simulink model "helicopter"  (R2024b)
settings: Solver=VariableStepAuto  StartTime=0.0  StopTime=60  RelTol=1e-3
InitFcn:
  | % run(fullfile(".\C:\Users\omar_\OneDrive - Imperial College London\EIE Year 4\FYP\model\controllers\controller_top"));
  | % run(fullfile(".\C:\Users\omar_\OneDrive - Imperial College London\EIE Year 4\FYP\model\helicopter_functions\R"));
  | % run(fullfile(".\C:\Users\omar_\OneDrive - Imperial College London\EIE Year 4\FYP\model\helicopter_functions\R_inv"));
  | % run(fullfile(".\C:\Users\omar_\OneDrive - Imperial College London\EIE Year 4\FYP\model\helicopter_functions\axial_thrust"));
  | % run(fullfile(".\C:\Users\omar_\OneDrive - Imperial College London\EIE Year 4\FYP\model\helicopter_functions\axial_thrust_bot"));
  | % run(fullfile(".\C:\Users\omar_\OneDrive - Imperial College London\EIE Year 4\FYP\model\helicopter_functions\axial_thrust_top"));
  | % run(fullfile(".\C:\Users\omar_\OneDrive - Imperial College London\EIE Year 4\FYP\model\helicopter_functions\body_update"));
  | % run(fullfile(".\C:\Users\omar_\OneDrive - Imperial College London\EIE Year 4\FYP\model\helicopter_functions\controller_top"));
  | % run(fullfile(".\C:\Users\omar_\OneDrive - Imperial College London\EIE Year 4\FYP\model\helicopter_functions\earth_update"));
  | % run(fullfile(".\C:\Users\omar_\OneDrive - Imperial College London\EIE Year 4\FYP\model\helicopter_functions\load_variables"));
  | % run(fullfile(".\C:\Users\omar_\OneDrive - Imperial College London\EIE Year 4\FYP\model\helicopter_functions\thrust_moments"));
  | % run(fullfile(".\C:\Users\omar_\OneDrive - Imperial College London\EIE Year 4\FYP\model\swash_plate\swash"));
  | % run(fullfile(".\C:\Users\omar_\OneDrive - Imperial College London\EIE Year 4\FYP\model\swash_plate\swash_height"));
  | rpm_top=300;
  | rpm_bot=300;
settings Model: Creator=omar_  LastModifiedBy=omar_
settings DataIOCC: ExternalInput=ext_sigs  LoadExternalInput=on

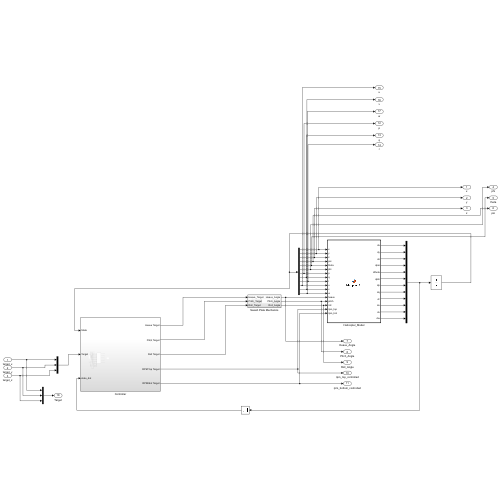
[thumbnail: Simulink's stored preview of the top-level diagram]
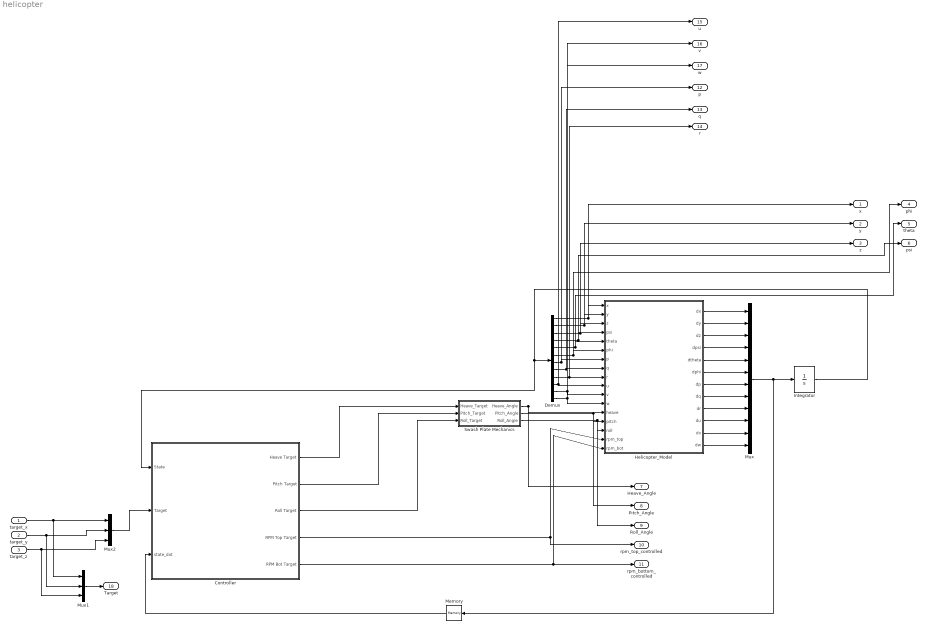
== system helicopter ==
  target_x : Inport
  target_y : Inport  Port=2
  target_z : Inport  Port=3
  Controller : Subsystem
  Demux : Demux  Outputs=12
  Helicopter_Model : MATLAB Function  TreatAsAtomicUnit=on
  Integrator : Integrator
  Memory : Memory
  Mux : Mux  Inputs=12
  Mux1 : Mux  Inputs=3
  Mux2 : Mux  Inputs=3
  Swash Plate Mechanics : Subsystem
  x : Outport
  y : Outport  Port=2
  z : Outport  Port=3
  phi : Outport  Port=4
  theta : Outport  Port=5
  psi : Outport  Port=6
  Heave_Angle : Outport  Port=7
  Pitch_Angle : Outport  Port=8
  Roll_Angle : Outport  Port=9
  rpm_top_controlled : Outport  Port=10
  rpm_bottom_controlled : Outport  Port=11
  p : Outport  Port=12
  q : Outport  Port=13
  r : Outport  Port=14
  u : Outport  Port=15
  v : Outport  Port=16
  w : Outport  Port=17
  Target : Outport  Port=18
  wires:
  Integrator/1 -> Demux/1, Controller/1(State)
  Demux/1 -> Helicopter_Model/1(x), x/1
  Demux/2 -> Helicopter_Model/2(y), y/1
  Demux/3 -> Helicopter_Model/3(z), z/1
  Demux/7 -> Helicopter_Model/7(p), p/1
  Demux/8 -> Helicopter_Model/8(q), q/1
  Demux/9 -> Helicopter_Model/9(r), r/1
  Demux/10 -> Helicopter_Model/10(u), u/1
  Demux/11 -> Helicopter_Model/11(v), v/1
  Demux/12 -> Helicopter_Model/12(w), w/1
  Helicopter_Model/1(dx) -> Mux/1
  Helicopter_Model/2(dy) -> Mux/2
  Helicopter_Model/3(dz) -> Mux/3
  Helicopter_Model/5(dtheta) -> Mux/5
  Helicopter_Model/7(dp) -> Mux/7
  Helicopter_Model/8(dq) -> Mux/8
  Helicopter_Model/9(dr) -> Mux/9
  Helicopter_Model/10(du) -> Mux/10
  Helicopter_Model/11(dv) -> Mux/11
  Helicopter_Model/12(dw) -> Mux/12
  Mux/1 -> Memory/1, Integrator/1
  Swash Plate Mechanics/1(Heave_Angle) -> Helicopter_Model/13(heave), Heave_Angle/1
  Demux/6 -> Helicopter_Model/6(phi), phi/1
  Demux/5 -> Helicopter_Model/5(theta), theta/1
  target_x/1 -> Mux2/1, Mux1/1
  target_y/1 -> Mux2/2, Mux1/2
  target_z/1 -> Mux2/3, Mux1/3
  Mux2/1 -> Controller/2(Target)
  Controller/4(RPM Top Target) -> Helicopter_Model/16(rpm_top), rpm_top_controlled/1
  Controller/5(RPM Bot Target) -> Helicopter_Model/17(rpm_bot), rpm_bottom_controlled/1
  Controller/1(Heave Target) -> Swash Plate Mechanics/1(Heave_Target)
  Controller/2(Pitch Target) -> Swash Plate Mechanics/2(Pitch_Target)
  Controller/3(Roll Target) -> Swash Plate Mechanics/3(Roll_Target)
  Memory/1 -> Controller/3(state_dot)
  Helicopter_Model/4(dpsi) -> Mux/4
  Helicopter_Model/6(dphi) -> Mux/6
  Demux/4 -> Helicopter_Model/4(psi), psi/1
  Swash Plate Mechanics/2(Pitch_Angle) -> Helicopter_Model/14(pitch), Pitch_Angle/1
  Swash Plate Mechanics/3(Roll_Angle) -> Roll_Angle/1, Helicopter_Model/15(roll)
  Mux1/1 -> Target/1

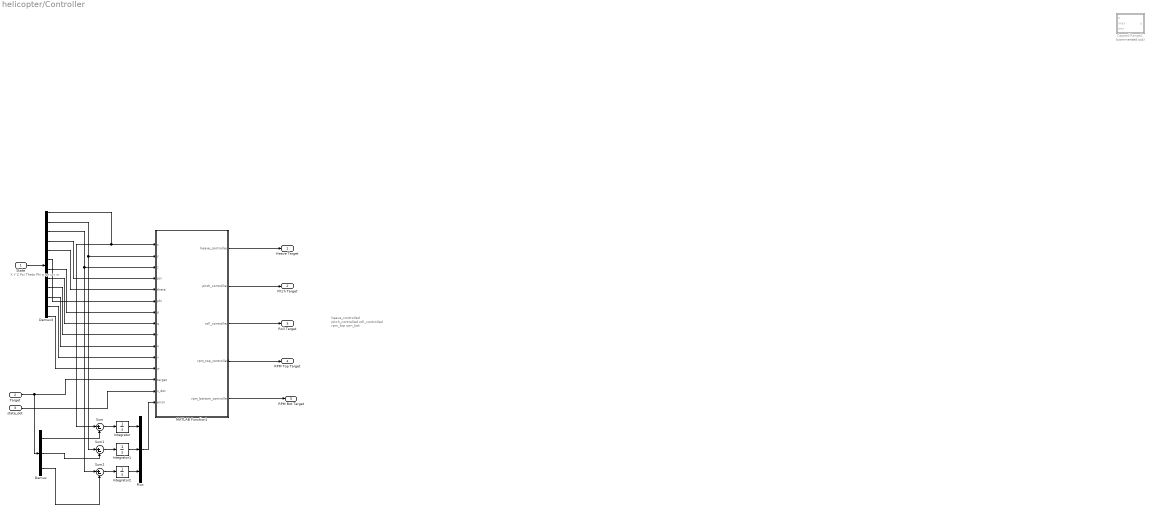
== system helicopter/Controller ==
  note: X
      | Y
      | Z
      | Psi
      | Theta
      | Phi
      | p
      | q
      | r
      | u
      | v
      | w
  note: heave_controlled
      | pitch_controlled
      | roll_controlled
      | rpm_top
      | rpm_bot
  State : Inport
  Target : Inport  Port=2
  state_dot : Inport  Port=3
  Capped Range1 : MATLAB Function  Commented=on  TreatAsAtomicUnit=on
  Demux : Demux  Outputs=3
  Demux3 : Demux  Outputs=12
  Integrator : Integrator
  Integrator1 : Integrator
  Integrator2 : Integrator
  MATLAB Function1 : MATLAB Function  TreatAsAtomicUnit=on
  Mux : Mux  Inputs=3
  Sum : Sum  Inputs=|+-
  Sum1 : Sum  Inputs=|+-
  Sum2 : Sum  Inputs=|+-
  Heave Target : Outport
  Pitch Target : Outport  Port=2
  Roll Target : Outport  Port=3
  RPM Top Target : Outport  Port=4
  RPM Bot Target : Outport  Port=5
  wires:
  Demux3/5 -> MATLAB Function1/5(theta)
  Demux3/3 -> MATLAB Function1/3(z), Sum2/1
  MATLAB Function1/3(roll_controlled) -> Roll Target/1
  Demux3/2 -> Sum1/1, MATLAB Function1/2(y)
  MATLAB Function1/5(rpm_bottom_controlled) -> RPM Bot Target/1
  MATLAB Function1/2(pitch_controlled) -> Pitch Target/1
  MATLAB Function1/1(heave_controlled) -> Heave Target/1
  MATLAB Function1/4(rpm_top_controlled) -> RPM Top Target/1
  Demux3/7 -> MATLAB Function1/7(p)
  Demux3/8 -> MATLAB Function1/8(q)
  Demux3/11 -> MATLAB Function1/11(v)
  Demux3/9 -> MATLAB Function1/9(r)
  Demux3/10 -> MATLAB Function1/10(u)
  Demux3/1 -> Sum/1, MATLAB Function1/1(x)
  Demux3/12 -> MATLAB Function1/12(w)
  State/1 -> Demux3/1
  state_dot/1 -> MATLAB Function1/14(x_dot)
  Target/1 -> Demux/1, MATLAB Function1/13(target)
  Sum/1 -> Integrator/1
  Sum1/1 -> Integrator1/1
  Sum2/1 -> Integrator2/1
  Demux/1 -> Sum/2
  Demux/2 -> Sum1/2
  Demux/3 -> Sum2/2
  Integrator/1 -> Mux/1
  Integrator1/1 -> Mux/2
  Integrator2/1 -> Mux/3
  Mux/1 -> MATLAB Function1/15(error)
  Demux3/4 -> MATLAB Function1/4(psi)
  Demux3/6 -> MATLAB Function1/6(phi)

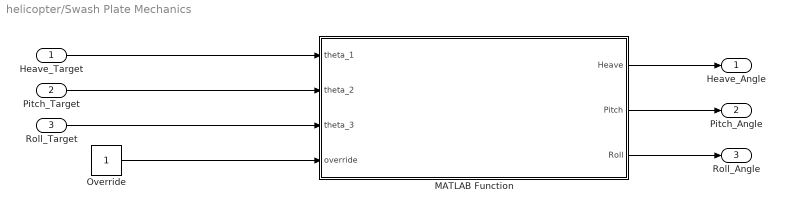
== system helicopter/Swash Plate Mechanics ==
  Heave_Target : Inport
  Pitch_Target : Inport  Port=2
  Roll_Target : Inport  Port=3
  MATLAB Function : MATLAB Function  TreatAsAtomicUnit=on
  Override : Constant
  Heave_Angle : Outport
  Pitch_Angle : Outport  Port=2
  Roll_Angle : Outport  Port=3
  wires:
  MATLAB Function/1(Heave) -> Heave_Angle/1
  MATLAB Function/2(Pitch) -> Pitch_Angle/1
  MATLAB Function/3(Roll) -> Roll_Angle/1
  Pitch_Target/1 -> MATLAB Function/2(theta_2)
  Roll_Target/1 -> MATLAB Function/3(theta_3)
  Heave_Target/1 -> MATLAB Function/1(theta_1)
  Override/1 -> MATLAB Function/4(override)

== matlab function helicopter/Controller/Capped Range1 ==
  data: u input; y output; max input; min input
function y = fcn(u, max, min)
    % disp(u)
    % disp(max)
    % if u >= min && u <= max
    % 
    %         y = u;
    % 
    % else
    % 
    %     if u <= min
    % 
    %         y = min;
    %     else
    %         y = max;
    %     end
    % 
    % end
    y = -0.2 + ((u - min) * 0.4) / (max - min);
    disp(y)

== matlab function helicopter/Swash Plate Mechanics/MATLAB Function ==
  data: theta_1 input double; Heave output double; theta_2 input double; theta_3 input double; Pitch output double; Roll output double; override input
function [Heave, Pitch, Roll] = Swash_Plate_Mechanics(theta_1, theta_2, theta_3, override)
    

    if override
        
        Heave = theta_1;
        Pitch = theta_2;
        Roll = theta_3;

    else
        variables = load("variables.mat", "rotation_plane_radius");
        heights = theta_to_h(theta_1, theta_2, theta_3);
        Heave = 1/3 * ( heights(1) + heights(2) + heights(3) );
        Pitch = asin( theta_1 / variables.rotation_plane_radius );
        Roll = 2;

    end

== matlab function helicopter/Helicopter_Model ==
  data: x input; y input; z input; psi input; theta input; phi input; p input; q input; r input; u input; dx output; dy output; dz output; dpsi output; dtheta output; dphi output; dp output; dq output; dr output; du output; dv output; dw output; v input; w input; heave input; pitch input; roll input; rpm_top input; rpm_bot input
function [dx,dy,dz,dpsi,dtheta,dphi,dp,dq,dr,du,dv,dw] = Helicopter_Top(x,y,z,psi,theta,phi,p,q,r,u,v,w,heave,pitch,roll,rpm_top,rpm_bot)
    result = body_update(x,y,z,psi,theta,phi,p,q,r,u,v,w,heave,pitch,roll,rpm_top,rpm_bot);
    
    dx     = result(1);
    dy     = result(2);
    dz     = result(3);
    dpsi   = result(4);
    dtheta = result(5);
    dphi   = result(6);
    dp     = result(7);
    dq     = result(8);
    dr     = result(9);
    du     = result(10);
    dv     = result(11);
    dw     = result(12);

== matlab function helicopter/Controller/MATLAB Function1 ==
  data: x input; y input; z input; psi input; theta input; phi input; p input; q input; r input; u input; heave_controlled output; v input; w input; target input; x_dot input; pitch_controlled output; roll_controlled output; rpm_top_controlled output; rpm_bottom_controlled output; error input
function [heave_controlled, pitch_controlled, roll_controlled, rpm_top_controlled, rpm_bottom_controlled] = controller_top(x,y,z,psi,theta,phi,p,q,r,u,v,w,target,x_dot,error)

    control_vector = controller(x,y,z,psi,theta,phi,p,q,r,u,v,w,target,x_dot,error);
    heave_controlled      = control_vector(1);
    pitch_controlled      = control_vector(2);
    roll_controlled       = control_vector(3);
    rpm_top_controlled    = control_vector(4);
    rpm_bottom_controlled = control_vector(5);
    % error                 = control_vector(6);
